simulink library "INT_CoTS_ThermDem"  (R2016b)
settings: Solver=VariableStepAuto  StartTime=0.0  StopTime=10.0  RelTol=1e-3
settings Model: Creator=xinchangran  LastModifiedBy=xinchangran

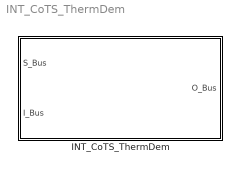
== system INT_CoTS_ThermDem ==
  INT_CoTS_ThermDem : Subsystem

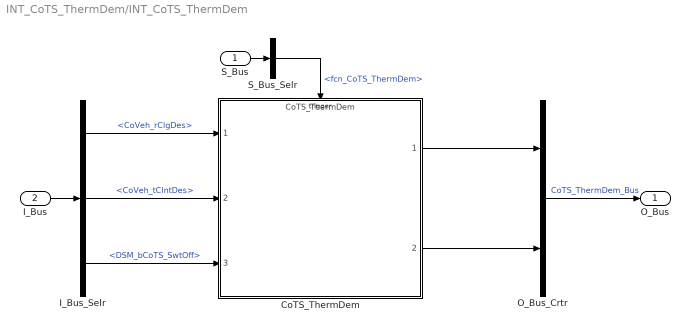
== system INT_CoTS_ThermDem/INT_CoTS_ThermDem ==
  S_Bus : Inport
  I_Bus : Inport  Port=2
  CoTS_ThermDem : ModelReference  ModelNameDialog=CoTS_ThermDem  SimulationMode=Normal  ModelReferenceVersion=1.29  TriggerPortName=function  TriggerPortTriggerType=function-call  TriggerPortStatesWhenEnabling=held
  I_Bus_Selr : BusSelector  OutputSignals=CoVeh_rClgDes,CoVeh_tClntDes,DSM_bCoTS_SwtOff
  O_Bus_Crtr : BusCreator  Inputs=2
  S_Bus_Selr : BusSelector  OutputSignals=fcn_CoTS_ThermDem
  O_Bus : Outport
  wires:
  S_Bus_Selr/1 -> CoTS_ThermDem/Trigger  "<fcn_CoTS_ThermDem>"
  S_Bus/1 -> S_Bus_Selr/1
  I_Bus/1 -> I_Bus_Selr/1
  I_Bus_Selr/1 -> CoTS_ThermDem/1  "<CoVeh_rClgDes>"
  I_Bus_Selr/2 -> CoTS_ThermDem/2  "<CoVeh_tClntDes>"
  I_Bus_Selr/3 -> CoTS_ThermDem/3  "<DSM_bCoTS_SwtOff>"
  O_Bus_Crtr/1 -> O_Bus/1  "CoTS_ThermDem_Bus"
  CoTS_ThermDem/1 -> O_Bus_Crtr/1
  CoTS_ThermDem/2 -> O_Bus_Crtr/2
